simulink model "Tanques_gravidade"  (R2021b)
settings: Solver=VariableStepAuto  StartTime=0.0  StopTime=Ts  RelTol=1e-3
InitFcn:
  | Ts = 25;
undefined symbols (not defined in the file or in its folder): input, volume_inicial
libraries: sh_lib x6, nesl_utility x4, fl_lib x2
settings Model: Creator=guilherme  LastModifiedBy=Gabri
settings SolverCC: MaxConsecutiveMinStep=2  AlgebraicLoopSolver=TrustRegion
settings DataIOCC: ReturnWorkspaceOutputs=off
settings DebuggingCC: SFMachineParentedDataDiag=warning  ArithmeticOperatorsInVariantConditions=warning
settings SFSimCC: SimUseLocalCustomCode=off  CustomCodeUndefinedFunction=UseInterfaceOnly
settings RTWCC: RTWUseLocalCustomCode=off
settings CodeAppCC: StateflowObjectComments=on
settings SimscapeCC: SimscapeNormalizeSystem=off

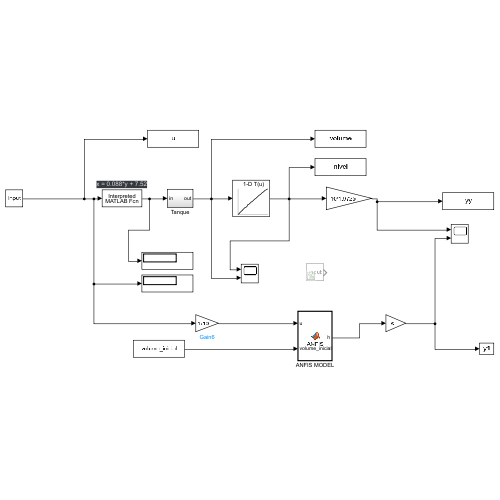
[thumbnail: Simulink's stored preview of the top-level diagram]
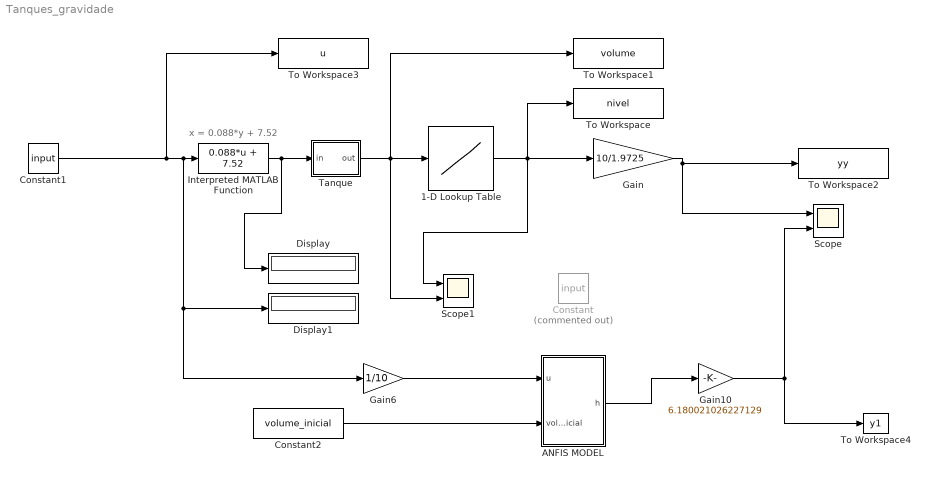
== system Tanques_gravidade ==
  note: x = 0.088*y + 7.52
  1-D Lookup Table : Lookup_n-D  NumberOfTableDimensions=1  BreakpointsForDimension1=[0, 0.0637, 0.1281, 0.1931, 0.2589, 0.3253, 0.3925, 0.4604, 0.5290, 0.5983, 0.6683, 0.7391, 0.8105, 0.8827, 0.9557, 1.0294, 1.1038, 1.1790, 1.2549, 1.3315, 1.4090, 1.4872, 1.5661, 1.6458, 1.7263, 1.8076, 1.8896, 1.9725]  Table=[0, 0.05, 0.1, 0.15, 0.2, 0.25, 0.3, 0.35, 0.4, 0.45, 0.5, 0.55, 0.6, 0.65, 0.7, 0.75, 0.8, 0.85, 0.9, 0.95, 1, 1.05, 1.1, 1.15, 1.2, 1.25, 1.3, 1.35]  InternalRulePriority=Speed  RndMeth=Simplest  InputSameDT=on
  ANFIS MODEL : MATLAB Function  TreatAsAtomicUnit=on
  Constant : Constant  Commented=on  Value=input
  Constant1 : Constant  Value=input
  Constant2 : Constant  Value=volume_inicial
  Display : Display
  Display1 : Display
  Gain : Gain  Gain=10/1.9725
  Gain10 : Gain  Gain=6.180021026227129
  Gain6 : Gain  Gain=1/10
  Interpreted MATLAB Function : MATLABFcn  MATLABFcn=0.088*u + 7.52  OutputDimensions=1
  Scope : Scope  NumInputPorts=2
  Scope1 : Scope  NumInputPorts=2
  Tanque : Subsystem
  To Workspace : ToWorkspace  VariableName=nivel  SampleTime=Ts
  To Workspace1 : ToWorkspace  VariableName=volume  SampleTime=Ts
  To Workspace2 : ToWorkspace  VariableName=yy  SampleTime=Ts
  To Workspace3 : ToWorkspace  VariableName=u  SampleTime=Ts
  To Workspace4 : ToWorkspace  VariableName=y1  SampleTime=Ts
  wires:
  1-D Lookup Table/1 -> Scope1/1, Gain/1, To Workspace/1
  Interpreted MATLAB Function/1 -> Display/1, Tanque/1(in)
  Gain/1 -> Scope/1, To Workspace2/1
  Gain6/1 -> ANFIS MODEL/1(u)
  Gain10/1 -> Scope/2, To Workspace4/1
  Constant1/1 -> Gain6/1, Display1/1, Interpreted MATLAB Function/1, To Workspace3/1
  ANFIS MODEL/1(h) -> Gain10/1
  Tanque/1(out) -> To Workspace1/1, Scope1/2, 1-D Lookup Table/1
  Constant2/1 -> ANFIS MODEL/2(volume_inicial)

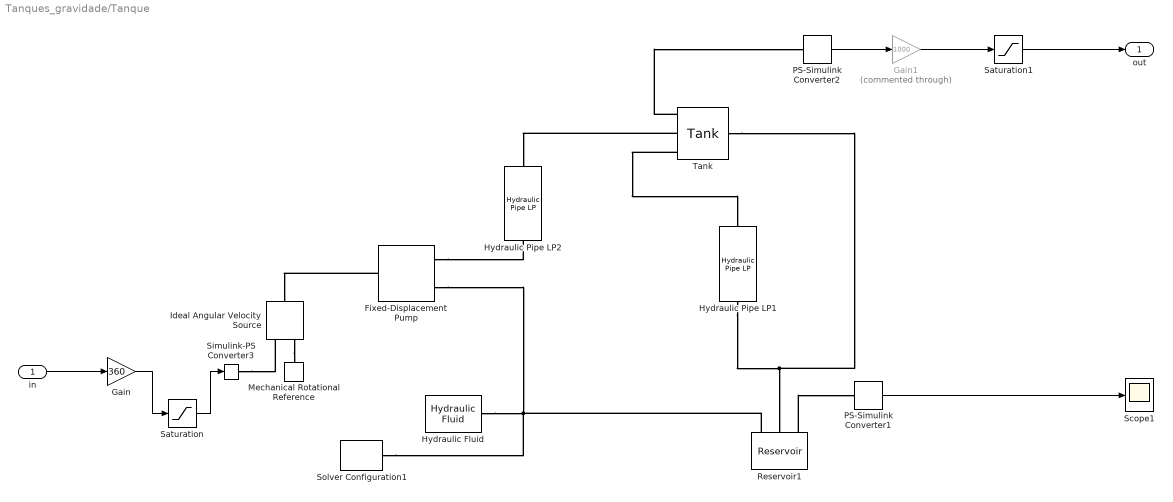
== system Tanques_gravidade/Tanque ==
  in : Inport
  Fixed-Displacement Pump : sh_lib/Pumps and Motors/Fixed-Displacement Pump  D=30 cm^3/rev  loss_spec=1  w_nominal=188 rad/s  pr_nominal=100e5 Pa  visc_nominal=18 cSt  dens_nominal=900 kg/m^3  efficiency_vol=0.92  no_load_torque=0.05 N*m  torque_pressure_coeff=0.6e-6 N*m/Pa  p_diff_eff_TLU=[100000, 1000000, 2000000] Pa  omega_eff_TLU=[25, 50, 100, 200, 300, 400] rad/s  vol_eff_TLU=[.816, .908, .954, .977, .981, .984; .325, .663, .831, .916, .925, .946; .137, .568, .78, .892, .893, .91]  mech_eff_TLU=[.996, .996, .996, .996, .996, .996; .988, .989, .989, .989, .989, .99; .981, .981, .982, .982, .983, .984]  p_diff_loss_TLU=[100000, 1000000, 2000000] Pa  omega_loss_TLU=[25, 50, 100, 200, 300, 400] rad/s  vol_loss_TLU=[.023, .023, .023, .023, .0285, .032; .0844, .0842, .0845, .084, .1125, .108; .1079, .108, .11, .108, .1605, .18] * 1e-3 m^3/s  mech_loss_TLU=[.002, .002, .002, .002, .002, .002; .0607, .0556, .0556, .0556, .0556, .0505; .1937, .1937, .1833, .1833, .1729, .1626] N*m  pressure_threshold=1e5 Pa  omega_threshold=10 rad/s  quadrant_check=0  pressure_check=0  min_valid_pressure=0 Pa  vol_eff_min=1e-3  vol_eff_max=1  mech_eff_min=1e-3  mech_eff_max=1
      settings: SourceProductBaseCode=SH  InternalSimscapePortConfiguration="{\"Bottom\":[],\"Left\":[{\"id\":\"S\",\"label\":\"S\",\"type\":\"foundation.mechanical.rotational.rotational\"}],\"Right\":[{\"id\":\"P\",\"label\":\"P\",\"type\":\"foundation.hydraulic.hydraulic\"},{\"id\":\"T\",\"label\":\"T\",\"type\":\"foundation.hydraulic.hydraulic\"}],\"Top\":[]}"
  Gain : Gain  Gain=360
  Gain1 : Gain  Commented=through  Gain=1000
  Hydraulic Fluid : sh_lib/Hydraulic Utilities/Hydraulic Fluid  DataSource=1  SelFluid=24  SysTemp=60  TrapAir=0.005  ViscDerFactor=1  range_error=2
  Hydraulic Pipe LP1 : sh_lib/Low-Pressure Blocks/Hydraulic Pipe LP  cs_type=1  d_in=53.35 mm  area=1e-4 m^2  D_h=1.12e-2 m  s_factor=64  length=5 m  length_ad=1 m  roughness=15e-6 m  Re_lam=2000  Re_turb=4000  p0=101325 Pa  wall_type=1  pr_r_coef=2e-12 m/Pa  time_const=0.01 s  k_sh=1.4  elevation_A=5 m  elevation_B=0 m  g=9.80665 m/s^2
      settings: SourceProductBaseCode=SH  InternalSimscapePortConfiguration="{\"Bottom\":[],\"Left\":[{\"id\":\"A\",\"label\":\"A\",\"type\":\"foundation.hydraulic.hydraulic\"}],\"Right\":[{\"id\":\"B\",\"label\":\"B\",\"type\":\"foundation.hydraulic.hydraulic\"}],\"Top\":[]}"
  Hydraulic Pipe LP2 : sh_lib/Low-Pressure Blocks/Hydraulic Pipe LP  cs_type=1  d_in=40 mm  area=1e-4 m^2  D_h=1.12e-2 m  s_factor=64  length=5 m  length_ad=1 m  roughness=15e-6 m  Re_lam=2000  Re_turb=4000  p0=101325 Pa  wall_type=1  pr_r_coef=2e-12 m/Pa  time_const=0.01 s  k_sh=1.4  elevation_A=6 m  elevation_B=1 m  g=9.80665 m/s^2
      settings: SourceProductBaseCode=SH  InternalSimscapePortConfiguration="{\"Bottom\":[],\"Left\":[{\"id\":\"A\",\"label\":\"A\",\"type\":\"foundation.hydraulic.hydraulic\"}],\"Right\":[{\"id\":\"B\",\"label\":\"B\",\"type\":\"foundation.hydraulic.hydraulic\"}],\"Top\":[]}"
  Ideal Angular Velocity Source : fl_lib/Mechanical/Mechanical Sources/Ideal Angular Velocity Source
  Mechanical Rotational Reference : fl_lib/Mechanical/Rotational Elements/Mechanical Rotational Reference
  PS-Simulink Converter1 : nesl_utility/PS-Simulink Converter  PhysicalDomain=network_engine_domain  SubClassName=ps_output  LeftPortType=input  RightPortType=output  PseudoPeriodic=off  Frequencies=[]  Unit=1  AffineConversion=off
      settings: SourceProductBaseCode=PW,SS
  PS-Simulink Converter2 : nesl_utility/PS-Simulink Converter  PhysicalDomain=network_engine_domain  SubClassName=ps_output  LeftPortType=input  RightPortType=output  PseudoPeriodic=off  Frequencies=[]  Unit=m^3  AffineConversion=off
      settings: SourceProductBaseCode=PW,SS
  Reservoir1 : sh_lib/Hydraulic Utilities/Reservoir  press=101325 Pa  init_volume=2000 l  ret_diam=1.5 in  loss_coeff=1
      settings: SourceProductBaseCode=SH  InternalSimscapePortConfiguration="{\"Bottom\":[],\"Left\":[{\"id\":\"V\",\"label\":\"V\",\"type\":\"output\"},{\"id\":\"P\",\"label\":\"P\",\"type\":\"foundation.hydraulic.hydraulic\"},{\"id\":\"R\",\"label\":\"R\",\"type\":\"foundation.hydraulic.hydraulic\"}],\"Right\":[],\"Top\":[]}"
  Saturation : Saturate  UpperLimit=3600  LowerLimit=750
  Saturation1 : Saturate  UpperLimit=inf  LowerLimit=0
  Scope1 : Scope
  Simulink-PS Converter3 : nesl_utility/Simulink-PS Converter  PhysicalDomain=network_engine_domain  SubClassName=ps_input  LeftPortType=input  RightPortType=output  PseudoPeriodic=off  Frequencies=[]  NoiseDistribution=none  NoiseParameters=[]  Unit=1  AffineConversion=off  FilteringAndDerivatives=provide  SimscapeFilterOrder=1  InputFilterTimeConstant=0.001  UdotUserProvided=0
      settings: SourceProductBaseCode=PW,SS
  Solver Configuration1 : nesl_utility/Solver Configuration  PhysicalDomain=network_engine_domain  SubClassName=solver  LeftPortType=input  RightPortType=generic  Tones=[]  Harmonics=[]  SimulateNoise=off  Profile=off  UseLocalSampling=off  EnableSwitchedLinearOptims=on  FrequencyDomain=off  UseCCode=off  RelTol=0.001  AbsTol=1e-06  MinStep=1e-09  ToWorkspace=off  RevertToSquareIcSolve=off  NumHomotopyIterations=100  PhasorMode=off  PhasorModeNumHarmonics=1  DoDC=off  ResidualTolerance=1e-09  UseLocalSolver=off  LocalSolverChoice=NE_BACKWARD_EULER_ADVANCER  LocalSolverSampleTime=0.001  DoFixedCost=off  MaxNonlinIter=3  MaxModeIter=2  ComputeImpulses=off  ImpulseIterations=2  LinearAlgebra=Sparse  EquationFormulation=NE_TIME_EF  DelaysMemoryBudget=1024  AutomaticFiltering=on  FilteringTimeConstant=0.001  PartitionStorageMethod=AS_NEEDED  PartitionMemoryBudget=1024  PartitionMethod=FAST
      settings: SourceProductBaseCode=PW,SS
  Tank : sh_lib/Low-Pressure Blocks/Tank  press=101325 Pa  level_spec=2  tank_area=1.7203 m^2  fluid_volume_tab=[0, 0.0637, 0.1281, 0.1931, 0.2589, 0.3253, 0.3925, 0.4604, 0.5290, 0.5983, 0.6683, 0.7391, 0.8105, 0.8827, 0.9557, 1.0294, 1.1038, 1.1790, 1.2549, 1.3315, 1.4090, 1.4872, 1.5661, 1.6458, 1.7263, 1.8076, 1.8896, 1.9725] m^3  fluid_level_tab=[0, 0.05, 0.1, 0.15, 0.2, 0.25, 0.3, 0.35, 0.4, 0.45, 0.5, 0.55, 0.6, 0.65, 0.7, 0.75, 0.8, 0.85, 0.9, 0.95, 1, 1.05, 1.1, 1.15, 1.2, 1.25, 1.3, 1.35] m  interp_method=2  extrap_method=1  pipe_diam=0.02 m  loss_coeff=1.2  g=9.80665 m/s^2  min_level=1e-3 m  fluid_level_check=0  volume_specify=on  volume_priority=High  volume=volume_inicial m^3  volume_nominal_specify=off  volume_nominal_unit=l  volume_nominal_value=1  level_specify=on  level_priority=None  level=0.1 m  level_nominal_specify=off  level_nominal_unit=m  level_nominal_value=1  pipe_diam_A=53.35 mm  loss_coeff_A=1.2  height_B=1 m  pipe_diam_B=40 mm  loss_coeff_B=1.2  height_C=1.35 m  pipe_diam_C=500 mm  loss_coeff_C=1.2
      settings: SourceProductBaseCode=SH  InternalSimscapePortConfiguration="{\"Bottom\":[],\"Left\":[{\"id\":\"V\",\"label\":\"V\",\"type\":\"output\"},{\"id\":\"B\",\"label\":\"B\",\"type\":\"foundation.hydraulic.hydraulic\"},{\"id\":\"A\",\"label\":\"A\",\"type\":\"foundation.hydraulic.hydraulic\"}],\"Right\":[{\"id\":\"C\",\"label\":\"C\",\"type\":\"foundation.hydraulic.hydraulic\"}],\"Top\":[]}"
  out : Outport
  wires:
  PS-Simulink Converter1/1 -> Scope1/1
  PS-Simulink Converter2/1 -> Gain1/1
  Gain1/1 -> Saturation1/1
  in/1 -> Gain/1
  Gain/1 -> Saturation/1
  Saturation/1 -> Simulink-PS Converter3/1
  Saturation1/1 -> out/1
  connections:
  Reservoir1/LConn1 -- PS-Simulink Converter1/LConn1
  Ideal Angular Velocity Source/RConn2 -- Mechanical Rotational Reference/LConn1
  Fixed-Displacement Pump/LConn1 -- Ideal Angular Velocity Source/LConn1
  Fixed-Displacement Pump/RConn1 -- Hydraulic Pipe LP2/RConn1
  Reservoir1/LConn3 -- Fixed-Displacement Pump/RConn2 -- Solver Configuration1/RConn1 -- Hydraulic Fluid/RConn1
  Hydraulic Pipe LP1/RConn1 -- Tank/RConn1 -- Reservoir1/LConn2
  Tank/LConn3 -- Hydraulic Pipe LP1/LConn1
  Simulink-PS Converter3/RConn1 -- Ideal Angular Velocity Source/RConn1
  Tank/LConn1 -- PS-Simulink Converter2/LConn1
  Tank/LConn2 -- Hydraulic Pipe LP2/LConn1

== matlab function Tanques_gravidade/ANFIS MODEL ==
  settings: updateMethod=DISCRETE  sampleTime=Ts
  data: u input; h output; volume_inicial input
function h = ANFIS(u, volume_inicial)
persistent b1 mean1 sigma1 ThetaL4 Mi NumInVars NumInTerms NumRules uo ho 

if isempty(Mi)
    uo = u;
    ho = volume_inicial;
    Mi          = 3;
    NumInVars   = Mi;
    NumInTerms  = 5;
    NumRules = NumInTerms;
    
    b1 = [-15.4759654931256,12.2209704903274,0.289123398113882,-71.9359064235566,21.1029827274901;53.1345392743568,59.6156777644246,24.2261619397451,-111.016028737690,-79.7593631490980;-27.2309348684618,-11.1514175692144,-0.889195034461636,12.4540272772075,30.5675786092304];
    mean1 = [-103.480659859437,0.160225765345676,47.1901134705417,55.2789314313193,493.802868016107;-101.143381316956,-86.2525384831843,-60.0254473600103,-49.3050420141232,61.7302726165688;-34.1633413139230,-17.2408154290438,-16.7182517919470,33.7842984316230,60.0187522106859];
    sigma1 = [75.1884591042617,-8.81165137905587,65.4355998025384,154.149488192979,19.3129732237862;-28.6583733437366,177.263377304061,-4.58534607185469,118.220932608957,-66.0488427183459;-104.852779993955,4.48200824012751,-18.0814276368059,51.2594822477457,13.0146519553683];
    ThetaL4 = [442.289967536936;-230.632389559791;-319.333734336911;-69.6453354552407;-0.0129190219528040;0.0350950739573748;0.977793760104156;-0.000167235344897465;-6655.46642722836;6554.95122169587;-448.603649444125;35.1420162336694;-1075.92572429594;1140.71744166750;-2455.19434546434;156.966414853777;109.045398229963;-80.6689421807745;9573.16412265227;-584.839849378831];
    h = ho;
    return
end
In1 = [uo; u; ho];

% LAYER 1 - INPUT TERM NODES
In2 = In1*ones(1,NumInTerms);
Out1 = 1./(1 + (abs((In2-mean1)./sigma1)).^(2*b1));

% LAYER 2 - PRODUCT NODES
Out2 = prod(Out1,1);
S_2 = sum(Out2);

% LAYER 3 - NORMALIZATION NODES
if S_2~=0
    Out3 = Out2'/S_2;
else
    Out3 = zeros(1,NumRules);
end

% LAYERS 4 - 5: CONSEQUENT NODES - SUMMING NODE
Aux1 = [In1; 1]*Out3';

% New Input Training Data shaped as a column vector.
a = reshape(Aux1,(NumInVars+1)*NumRules,1);

h_a = a'*ThetaL4;

ho = h_a;
uo = u;

h = h_a;
